simulink model "async_flier_modelling_non_d"  (R2023a)
settings: Solver=VariableStepAuto  StartTime=0.0  StopTime=2000  FixedStep=dt  MaxStep=dt  RelTol=1e-6
values from neighbouring files (symbols this model uses):
  kd = 0.5    [Find_Lambda_F_by_K_diff_amp_async.m]    (also in Find_Lamda_F_by_K_async.m; Find_Lamda_F_by_K_sync.m)
  kt = 1 - ku - kd    (= 0)    [Find_Lambda_F_by_K_diff_amp_async.m]    (also in Find_Lamda_F_by_K_async.m; Find_Lamda_F_by_K_sync.m)
  ku = 0.5    [Find_Lambda_F_by_K_diff_amp_async.m]    (also in Find_Lamda_F_by_K_async.m; Find_Lamda_F_by_K_sync.m)
  P1 = P1allnew(1,p1i)    [Find_Lambda_F_by_K_diff_amp_async.m]    (also in Find_Lamda_F_by_K_async.m; Find_Lamda_F_by_K_sync.m = P1allfinal(1,p1i); Find_Lamda_F_by_K_sync_no_spring.m = P1allfinal(1,p1i))
  P2 = P2 + 0.05    [Find_Lambda_F_by_K_diff_amp_async.m]    (also in Find_Lamda_F_by_K_async.m = 0.1; Find_Lamda_F_by_K_sync.m = P2new(1,p1i-1); Find_Lamda_F_by_K_sync_no_spring.m = P2new(1,p1i-1))
  t0 = 0.5    [Find_Lambda_F_by_K_diff_amp_async.m]    (also in Find_Lamda_F_by_K_async.m)
  xt = 0    [Find_Lambda_F_by_K_diff_amp_async.m]    (also in Find_Lamda_F_by_K_async.m; Find_Lamda_F_by_K_sync.m)
undefined symbols (not defined in the file or in its folder): a1, a2, a3, mu
libraries: simulink x12
settings Model: Creator=suyash  LastModifiedBy=suyash
settings DebuggingCC: UnconnectedInputMsg=warning  UnconnectedOutputMsg=warning  UnconnectedLineMsg=warning
settings ModelReferenceCC: EnableRefExpFcnMdlSchedulingChecks=on
settings RTWCC: DLArmComputeVersion=19.05

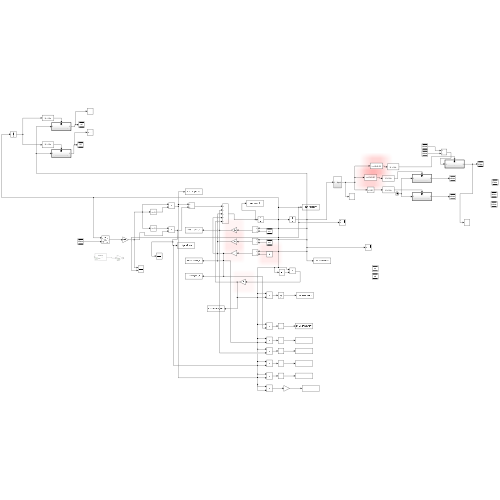
[thumbnail: Simulink's stored preview of the top-level diagram]
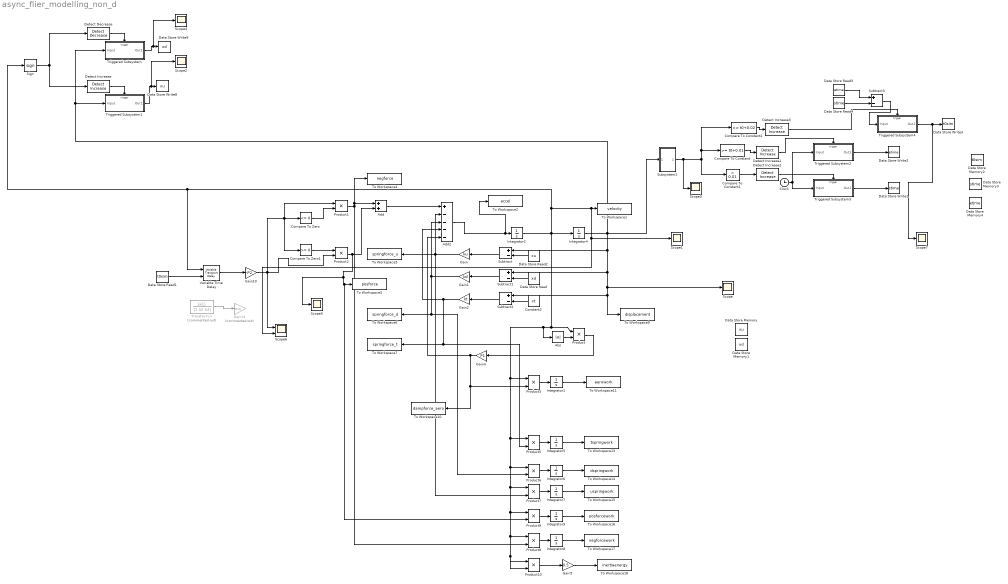
== system async_flier_modelling_non_d ==
  Abs : Abs  SaturateOnIntegerOverflow=off
  Add : Sum
  Add2 : Sum  Inputs=+----
  Clock : Clock
  Compare To Constant : simulink/Logic and Bit Operations/Compare To Constant  relop=>=  const=t0+0.01  OutDataTypeStr=boolean
  Compare To Constant1 : simulink/Logic and Bit Operations/Compare To Constant  relop=>  const=0.01  OutDataTypeStr=boolean
  Compare To Constant2 : simulink/Logic and Bit Operations/Compare To Constant  relop=>=  const=t0+0.02  OutDataTypeStr=boolean
  Compare To Zero : simulink/Logic and Bit Operations/Compare To Zero  relop=<=  OutDataTypeStr=boolean
  Compare To Zero1 : simulink/Logic and Bit Operations/Compare To Zero  relop=>=  OutDataTypeStr=boolean
  Constant2 : Constant  Value=xt
  Data Store Memory : DataStoreMemory  DataStoreName=xu  ReadBeforeWriteMsg=warning  WriteAfterWriteMsg=warning  WriteAfterReadMsg=warning  ShowAdditionalParam=off
  Data Store Memory1 : DataStoreMemory  DataStoreName=xd  ReadBeforeWriteMsg=warning  WriteAfterWriteMsg=warning  WriteAfterReadMsg=warning  ShowAdditionalParam=off
  Data Store Memory2 : DataStoreMemory  DataStoreName=t0sim  ReadBeforeWriteMsg=warning  WriteAfterWriteMsg=warning  WriteAfterReadMsg=warning  ShowAdditionalParam=off
  Data Store Memory3 : DataStoreMemory  DataStoreName=stime  ReadBeforeWriteMsg=warning  WriteAfterWriteMsg=warning  WriteAfterReadMsg=warning  ShowAdditionalParam=off
  Data Store Memory4 : DataStoreMemory  DataStoreName=etime  ReadBeforeWriteMsg=warning  WriteAfterWriteMsg=warning  WriteAfterReadMsg=warning  ShowAdditionalParam=off
  Data Store Read : DataStoreRead  DataStoreName=xd  IndexOptions=Index vector (dialog)  Indices=1  OutputSizes=1
  Data Store Read1 : DataStoreRead  DataStoreName=t0sim  IndexOptions=Index vector (dialog)  Indices=1  OutputSizes=1
  Data Store Read2 : DataStoreRead  DataStoreName=xu  IndexOptions=Index vector (dialog)  Indices=1  OutputSizes=1
  Data Store Read3 : DataStoreRead  DataStoreName=etime  IndexOptions=Index vector (dialog)  Indices=1  OutputSizes=1
  Data Store Read4 : DataStoreRead  DataStoreName=stime  IndexOptions=Index vector (dialog)  Indices=1  OutputSizes=1
  Data Store Write1 : DataStoreWrite  DataStoreName=stime  IndexOptions=Index vector (dialog)  Indices=1  OutputSizes=1
  Data Store Write2 : DataStoreWrite  DataStoreName=etime  IndexOptions=Index vector (dialog)  Indices=1  OutputSizes=1
  Data Store Write3 : DataStoreWrite  DataStoreName=t0sim  IndexOptions=Index vector (dialog)  Indices=1  OutputSizes=1
  Data Store Write8 : DataStoreWrite  DataStoreName=xu  IndexOptions=Index vector (dialog)  Indices=1  OutputSizes=1
  Data Store Write9 : DataStoreWrite  DataStoreName=xd  IndexOptions=Index vector (dialog)  Indices=1  OutputSizes=1
  Detect Decrease : simulink/Logic and Bit Operations/Detect Decrease  vinit=0.0  OutDataTypeStr=boolean
  Detect Increase{,1..3} (4 alike) : simulink/Logic and Bit Operations/Detect Increase  vinit=0.0  OutDataTypeStr=boolean
  Gain : Gain  Gain=ku
  Gain1 : Gain  Gain=kd
  Gain10 : Gain  Gain=-P2
  Gain14 : Gain  Commented=on  Gain=mu
  Gain2 : Gain  Gain=kt
  Gain4 : Gain  Gain=P1
  Gain5 : Gain  Gain=0.5
  Integrator{1,4..9} (7 alike) : Integrator
  Integrator2 : Integrator  InitialCondition=0.1
  Product{,1..3,5..10} (10 alike) : Product
  Scope{,1..5,7} (7 alike) : Scope
  Scope6 : Scope  NumInputPorts=2
  Sign : Signum
  Subsystem2 : Subsystem
  Subtract{,1..3} (4 alike) : Sum  Inputs=+-
  To Workspace1 : ToWorkspace  VariableName=velocity  SaveFormat=Timeseries  SampleTime=-1
  To Workspace10 : ToWorkspace  VariableName=dampforce_aero  SaveFormat=Timeseries  SampleTime=-1
  To Workspace11 : ToWorkspace  VariableName=aerowork  SaveFormat=Timeseries  SampleTime=-1
  To Workspace13 : ToWorkspace  VariableName=tspringwork  SaveFormat=Timeseries  SampleTime=-1
  To Workspace14 : ToWorkspace  VariableName=dspringwork  SaveFormat=Timeseries  SampleTime=-1
  To Workspace15 : ToWorkspace  VariableName=uspringwork  SaveFormat=Timeseries  SampleTime=-1
  To Workspace16 : ToWorkspace  VariableName=posforcework  SaveFormat=Timeseries  SampleTime=-1
  To Workspace17 : ToWorkspace  VariableName=negforcework  SaveFormat=Timeseries  SampleTime=-1
  To Workspace18 : ToWorkspace  VariableName=inertiaenergy  SaveFormat=Timeseries  SampleTime=-1
  To Workspace2 : ToWorkspace  VariableName=accel  SaveFormat=Timeseries  SampleTime=-1
  To Workspace3 : ToWorkspace  VariableName=posforce  SaveFormat=Timeseries  SampleTime=-1
  To Workspace4 : ToWorkspace  VariableName=negforce  SaveFormat=Timeseries  SampleTime=-1
  To Workspace5 : ToWorkspace  VariableName=springforce_u  SaveFormat=Timeseries  SampleTime=-1
  To Workspace6 : ToWorkspace  VariableName=springforce_d  SaveFormat=Timeseries  SampleTime=-1
  To Workspace7 : ToWorkspace  VariableName=springforce_t  SaveFormat=Timeseries  SampleTime=-1
  To Workspace9 : ToWorkspace  VariableName=displacement  SaveFormat=Timeseries  SampleTime=-1
  Transfer Fcn : TransferFcn  Commented=on  Numerator=[a1]  Denominator=[1 a2 a3]
  Triggered Subsystem : Subsystem  TreatAsAtomicUnit=on
  Triggered Subsystem1 : Subsystem  TreatAsAtomicUnit=on
  Triggered Subsystem2 : Subsystem  TreatAsAtomicUnit=on
  Triggered Subsystem3 : Subsystem  TreatAsAtomicUnit=on
  Triggered Subsystem4 : Subsystem  TreatAsAtomicUnit=on
  Variable Time Delay : VariableTransportDelay  MaximumDelay=10
  wires:
  Add2/1 -> To Workspace2/1, Integrator2/1
  Data Store Read2/1 -> Subtract/2
  Subtract/1 -> Gain/1
  Gain/1 -> Product7/2, To Workspace5/1, Add2/2
  Subtract1/1 -> Gain1/1
  Data Store Read/1 -> Subtract1/2
  Subtract2/1 -> Gain2/1
  Constant2/1 -> Subtract2/2
  Gain1/1 -> Product6/2, To Workspace6/1, Add2/3
  Gain2/1 -> To Workspace7/1, Product5/2, Add2/4
  Product/1 -> Gain4/1
  Gain4/1 -> To Workspace10/1, Product3/2, Add2/5
  Abs/1 -> Product/2
  Add/1 -> Add2/1
  Compare To Zero/1 -> Product1/2
  Compare To Zero1/1 -> Product2/1
  Product2/1 -> Scope5/1, Product9/2, To Workspace3/1, Add/2
  Product1/1 -> To Workspace4/1, Add/1, Product8/2
  Variable Time Delay/1 -> Gain10/1
  Gain10/1 -> Scope6/1, Compare To Zero1/1, Compare To Zero/1, Product1/1, Product2/2
  Product6/1 -> Integrator6/1
  Product5/1 -> Integrator5/1
  Integrator7/1 -> To Workspace15/1
  Product10/1 -> Gain5/1
  Gain5/1 -> To Workspace18/1
  Integrator6/1 -> To Workspace14/1
  Integrator8/1 -> To Workspace17/1
  Product3/1 -> Integrator1/1
  Integrator9/1 -> To Workspace16/1
  Product7/1 -> Integrator7/1
  Product8/1 -> Integrator8/1
  Product9/1 -> Integrator9/1
  Integrator5/1 -> To Workspace13/1
  Integrator1/1 -> To Workspace11/1
  Triggered Subsystem1/1(Out1) -> Scope2/1, Data Store Write8/1
  Triggered Subsystem/1(Out1) -> Scope4/1, Data Store Write9/1
  Detect Decrease/1 -> Triggered Subsystem/Trigger
  Sign/1 -> Detect Increase/1, Detect Decrease/1
  Detect Increase/1 -> Triggered Subsystem1/Trigger
  Integrator2/1 -> Variable Time Delay/1, Sign/1, Scope6/2, Scope1/1, To Workspace1/1, Product10/2, Product10/1, Product8/1, Product9/1, Product7/1, Product6/1, Product5/1, Product3/1, Abs/1, Product/1, Integrator4/1
  Transfer Fcn/1 -> Gain14/1
  Integrator4/1 -> Subsystem2/1(In1), Scope/1, To Workspace9/1, Subtract2/1, Subtract1/1, Subtract/1, Triggered Subsystem1/1(Input), Triggered Subsystem/1(Input)
  Triggered Subsystem3/1(Out1) -> Data Store Write1/1
  Clock/1 -> Triggered Subsystem3/1(Input), Triggered Subsystem2/1(Input)
  Subtract3/1 -> Triggered Subsystem4/1(Input)
  Subsystem2/1(Input) -> Scope3/1, Compare To Constant1/1, Compare To Constant2/1, Compare To Constant/1
  Compare To Constant/1 -> Detect Increase1/1
  Data Store Read3/1 -> Subtract3/1
  Detect Increase2/1 -> Triggered Subsystem3/Trigger
  Triggered Subsystem2/1(Out1) -> Data Store Write2/1
  Compare To Constant2/1 -> Detect Increase3/1
  Detect Increase3/1 -> Triggered Subsystem4/Trigger
  Detect Increase1/1 -> Triggered Subsystem2/Trigger
  Data Store Read4/1 -> Subtract3/2
  Compare To Constant1/1 -> Detect Increase2/1
  Triggered Subsystem4/1(Out1) -> Scope7/1, Data Store Write3/1
  Data Store Read1/1 -> Variable Time Delay/2

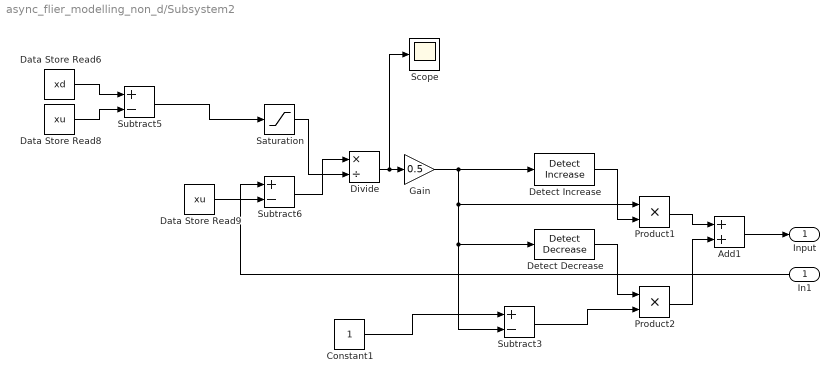
== system async_flier_modelling_non_d/Subsystem2 ==
  In1 : Inport
  Add1 : Sum
  Constant1 : Constant
  Data Store Read6 : DataStoreRead  DataStoreName=xd  IndexOptions=Index vector (dialog)  Indices=1  OutputSizes=1
  Data Store Read8 : DataStoreRead  DataStoreName=xu  IndexOptions=Index vector (dialog)  Indices=1  OutputSizes=1
  Data Store Read9 : DataStoreRead  DataStoreName=xu  IndexOptions=Index vector (dialog)  Indices=1  OutputSizes=1
  Detect Decrease : simulink/Logic and Bit Operations/Detect Decrease  vinit=0.0  OutDataTypeStr=boolean
  Detect Increase : simulink/Logic and Bit Operations/Detect Increase  vinit=0.0  OutDataTypeStr=boolean
  Divide : Product  Inputs=*/
  Gain : Gain  Gain=0.5
  Product1 : Product
  Product2 : Product
  Saturation : Saturate  UpperLimit=100  LowerLimit=0.01
  Scope : Scope
  Subtract3 : Sum  Inputs=+-
  Subtract5 : Sum  Inputs=+-
  Subtract6 : Sum  Inputs=+-
  Input : Outport
  wires:
  Subtract3/1 -> Product2/2
  Product2/1 -> Add1/2
  Constant1/1 -> Subtract3/1
  Add1/1 -> Input/1
  Subtract6/1 -> Divide/1
  Data Store Read9/1 -> Subtract6/2
  Data Store Read6/1 -> Subtract5/1
  Data Store Read8/1 -> Subtract5/2
  Detect Decrease/1 -> Product2/1
  In1/1 -> Subtract6/1
  Divide/1 -> Scope/1, Gain/1
  Product1/1 -> Add1/1
  Detect Increase/1 -> Product1/2
  Gain/1 -> Detect Increase/1, Detect Decrease/1, Subtract3/2, Product1/1
  Subtract5/1 -> Saturation/1
  Saturation/1 -> Divide/2

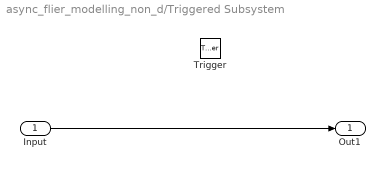
== system async_flier_modelling_non_d/Triggered Subsystem ==
  Input : Inport
  Trigger : TriggerPort  VariantControl=(inherit)
  Out1 : Outport
  wires:
  Input/1 -> Out1/1

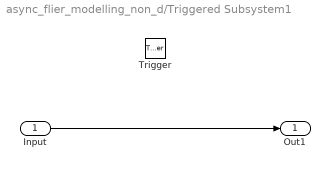
== system async_flier_modelling_non_d/Triggered Subsystem1 ==
  Input : Inport
  Trigger : TriggerPort  VariantControl=(inherit)
  Out1 : Outport
  wires:
  Input/1 -> Out1/1

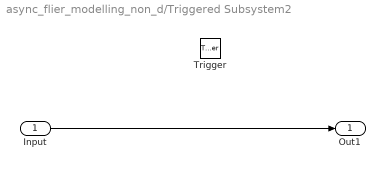
== system async_flier_modelling_non_d/Triggered Subsystem2 ==
  Input : Inport
  Trigger : TriggerPort  VariantControl=(inherit)
  Out1 : Outport
  wires:
  Input/1 -> Out1/1

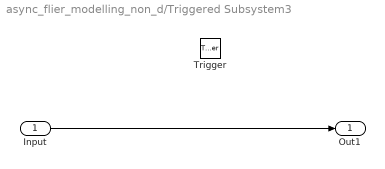
== system async_flier_modelling_non_d/Triggered Subsystem3 ==
  Input : Inport
  Trigger : TriggerPort  VariantControl=(inherit)
  Out1 : Outport
  wires:
  Input/1 -> Out1/1

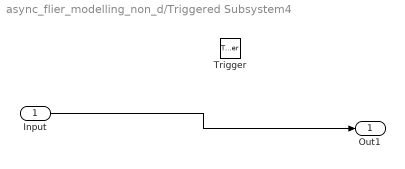
== system async_flier_modelling_non_d/Triggered Subsystem4 ==
  Input : Inport
  Trigger : TriggerPort  VariantControl=(inherit)
  Out1 : Outport
  wires:
  Input/1 -> Out1/1
